simulink model "sim1"  (R2023a)
settings: Solver=VariableStepAuto  StartTime=0  StopTime=19  RelTol=1e-8
undefined symbols (not defined in the file): a0, a1, a2, k0, k1, T
settings Model: Creator=vasil  LastModifiedBy=vasil

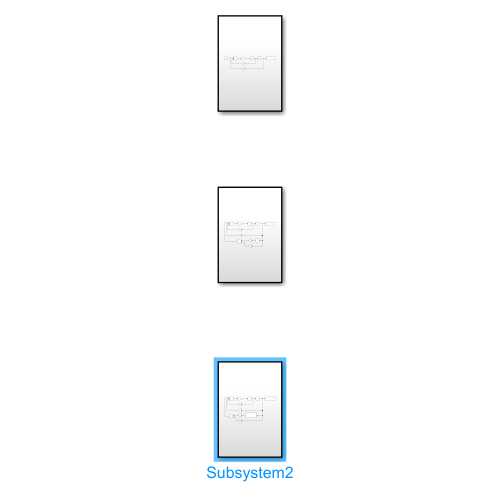
[thumbnail: Simulink's stored preview of the top-level diagram]
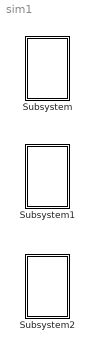
== system sim1 ==
  Subsystem : Subsystem
  Subsystem1 : Subsystem
  Subsystem2 : Subsystem

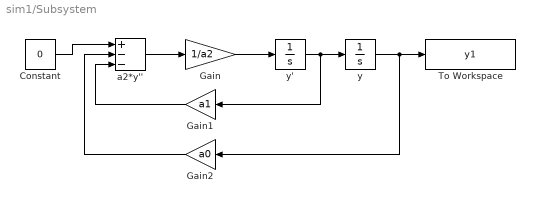
== system sim1/Subsystem ==
  Constant : Constant  Value=0
  Gain : Gain  Gain=1/a2
  Gain1 : Gain  Gain=a1
  Gain2 : Gain  Gain=a0
  To Workspace : ToWorkspace  VariableName=y1  SaveFormat=Timeseries  SampleTime=-1
  a2*y'' : Sum  Inputs=+--
  y : Integrator
  y' : Integrator  InitialCondition=1
  wires:
  y'/1 -> Gain1/1, y/1
  y/1 -> Gain2/1, To Workspace/1
  Gain1/1 -> a2*y''/3
  Gain2/1 -> a2*y''/2
  Constant/1 -> a2*y''/1
  a2*y''/1 -> Gain/1
  Gain/1 -> y'/1

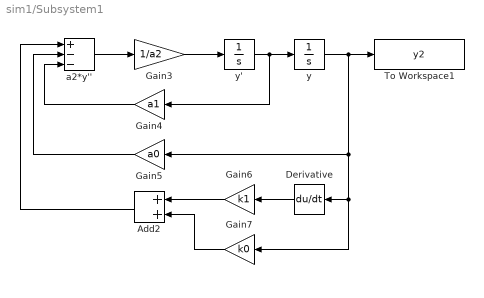
== system sim1/Subsystem1 ==
  Add2 : Sum
  Derivative : Derivative
  Gain3 : Gain  Gain=1/a2
  Gain4 : Gain  Gain=a1
  Gain5 : Gain  Gain=a0
  Gain6 : Gain  Gain=k1
  Gain7 : Gain  Gain=k0
  To Workspace1 : ToWorkspace  VariableName=y2  SaveFormat=Timeseries  SampleTime=-1
  a2*y'' : Sum  Inputs=+--
  y : Integrator
  y' : Integrator  InitialCondition=1
  wires:
  Gain7/1 -> Add2/2
  Add2/1 -> a2*y''/1
  Gain6/1 -> Add2/1
  y/1 -> Gain7/1, Derivative/1, Gain5/1, To Workspace1/1
  Gain3/1 -> y'/1
  Gain4/1 -> a2*y''/3
  a2*y''/1 -> Gain3/1
  y'/1 -> Gain4/1, y/1
  Derivative/1 -> Gain6/1
  Gain5/1 -> a2*y''/2

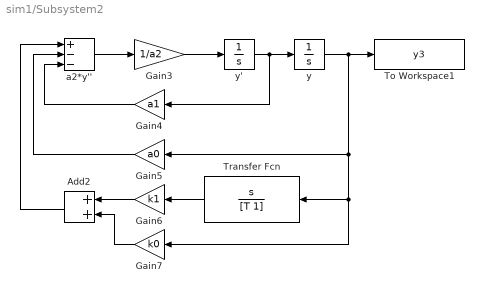
== system sim1/Subsystem2 ==
  Add2 : Sum
  Gain3 : Gain  Gain=1/a2
  Gain4 : Gain  Gain=a1
  Gain5 : Gain  Gain=a0
  Gain6 : Gain  Gain=k1
  Gain7 : Gain  Gain=k0
  To Workspace1 : ToWorkspace  VariableName=y3  SaveFormat=Timeseries  SampleTime=-1
  Transfer Fcn : TransferFcn  Numerator=[1 0]  Denominator=[T 1]
  a2*y'' : Sum  Inputs=+--
  y : Integrator
  y' : Integrator  InitialCondition=1
  wires:
  Gain6/1 -> Add2/1
  Gain3/1 -> y'/1
  y/1 -> Gain7/1, Transfer Fcn/1, Gain5/1, To Workspace1/1
  Gain5/1 -> a2*y''/2
  y'/1 -> Gain4/1, y/1
  Gain4/1 -> a2*y''/3
  a2*y''/1 -> Gain3/1
  Add2/1 -> a2*y''/1
  Gain7/1 -> Add2/2
  Transfer Fcn/1 -> Gain6/1
